simulink library "csc_estimation_lib"  (R2015b)
settings: Solver=ode45  StartTime=0.0  StopTime=10.0  RelTol=1e-3
undefined symbols (not defined in the file): csu_kfo_kalman_filter_output, csu_kfo_kalman_filter_output_lib, est_time_step
libraries: util_info_lib x4, util_common_lib x4, csc_emp_est_mass_props_lib x2, csc_kfl_kalman_filter_lib x2, csc_spc_sensor_processing_lib x2, csu_elk_est_landed_kinematics_lib x2, csu_esf_est_switch_frame_lib x2, util_frame_rotation_lib x2
settings Model: Creator=ianmga  LastModifiedBy=Mark Agbayani
settings DataIOCC: SaveFormat=Array  SignalLoggingSaveFormat=ModelDataLogs
settings OptimizationCC: ExpressionDepthLimit=2147483647
settings DebuggingCC: UnderspecifiedInitializationDetection=Classic  MergeDetectMultiDrivingBlocksExec=none  SolverPrmCheckMsg=warning  FcnCallInpInsideContextMsg=UseLocalSettings  StateNameClashWarn=warning
settings HardwareCC: ProdBitPerPointer=32  ProdLargestAtomicFloat=None  ProdIntDivRoundTo=Undefined  ProdEndianess=Unspecified  ProdWordSize=32  ProdHWDeviceType=32-bit Generic
settings GRTTargetCC: GeneratePreprocessorConditionals=Disable all  CombineOutputUpdateFcns=off  GRTInterface=on
settings ConfigComp: CovModelRefEnable=Off  CovSFcnEnable=off

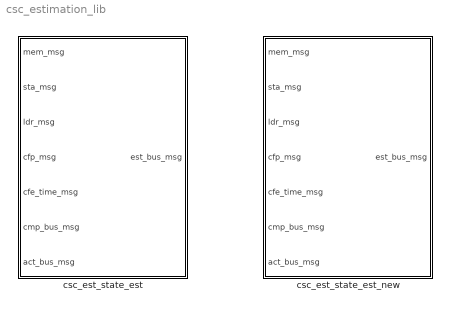
== system csc_estimation_lib ==
  csc_est_state_est : Subsystem  Tag=OFSW; MDL_TICK=CMP_BUS_MSG  TreatAsAtomicUnit=on  SystemSampleTime=est_time_step
  csc_est_state_est_new : Subsystem  Tag=OFSW; MDL_TICK=CMP_BUS_MSG  TreatAsAtomicUnit=on  SystemSampleTime=est_time_step

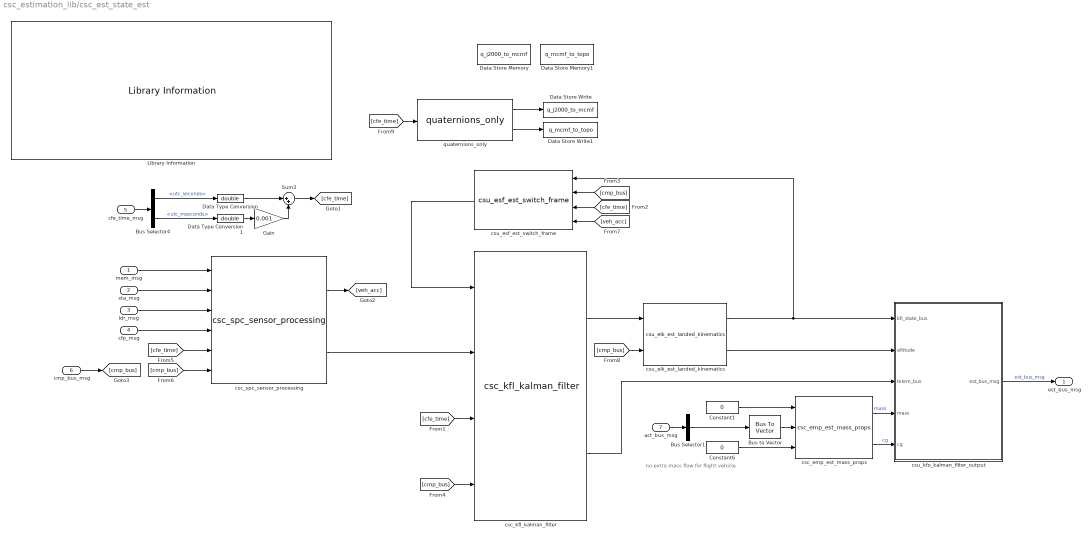
== system csc_estimation_lib/csc_est_state_est ==
  note: no extra mass flow for flight vehicle
  mem_msg : Inport  OutDataTypeStr=Bus: mem_msg
  sta_msg : Inport  Port=2  OutDataTypeStr=Bus: sta_msg
  ldr_msg : Inport  Port=3  OutDataTypeStr=Bus: ldr_msg
  cfp_msg : Inport  Port=4  OutDataTypeStr=Bus: cfp_msg
  cfe_time_msg : Inport  Port=5  OutDataTypeStr=Bus: cfe_time_msg
  cmp_bus_msg : Inport  Port=6  OutDataTypeStr=Bus: cmp_bus_msg
  act_bus_msg : Inport  Port=7  OutDataTypeStr=Bus: act_bus_msg
  Bus Selector1 : BusSelector  OutputSignals=coarse1_time,coarse2_time,coarse3_time,coarse4_time,coarse5_time,coarse6_time,coarse7_time,coarse8_time,coarse9_time,coarse10_time,coarse11_time,coarse12_time,fine1_time,fine2_time,fine3_time,fine4_time,fine5_time,fine6_time,fine7_time,fine8_time,fine9_time,fine10_time,fine11_time,fine12_time,main_thruster_cmd,main_biprop_monoprop  OutputAsBus=on
  Bus Selector4 : BusSelector  OutputSignals=utc_seconds,utc_mseconds
  Bus to Vector : BusToVector
  Constant1 : Constant  Value=0
  Constant6 : Constant  Value=0
  Data Store Memory : DataStoreMemory  DataStoreName=q_j2000_to_mcmf  ReadBeforeWriteMsg=warning  WriteAfterWriteMsg=warning  WriteAfterReadMsg=warning  InitialValue=[0 0 0 1]  OutDataTypeStr=double
  Data Store Memory1 : DataStoreMemory  DataStoreName=q_mcmf_to_topo  ReadBeforeWriteMsg=warning  WriteAfterWriteMsg=warning  WriteAfterReadMsg=warning  InitialValue=[0 0 0 1]  OutDataTypeStr=double
  Data Store Write : DataStoreWrite  DataStoreName=q_j2000_to_mcmf
  Data Store Write1 : DataStoreWrite  DataStoreName=q_mcmf_to_topo
  Data Type Conversion : DataTypeConversion  OutDataTypeStr=double
  Data Type Conversion1 : DataTypeConversion  OutDataTypeStr=double
  Gain : Gain  Gain=0.001
  Library Information : util_info_lib/Library Information  owner='NONE'
  Sum2 : Sum  Inputs=|++
  csc_emp_est_mass_props : csc_emp_est_mass_props_lib/csc_emp_est_mass_props
  csc_kfl_kalman_filter : csc_kfl_kalman_filter_lib/csc_kfl_kalman_filter
  csc_spc_sensor_processing : csc_spc_sensor_processing_lib/csc_spc_sensor_processing
  csu_elk_est_landed_kinematics : csu_elk_est_landed_kinematics_lib/csu_elk_est_landed_kinematics
  csu_esf_est_switch_frame : csu_esf_est_switch_frame_lib/csu_esf_est_switch_frame
  csu_kfo_kalman_filter_output : Subsystem  AncestorBlock=csu_kfo_kalman_filter_output_lib/csu_kfo_kalman_filter_output
  quaternions_only : util_frame_rotation_lib/quaternions_only  SystemSampleTime=-1
  est_bus_msg : Outport  OutDataTypeStr=Bus: est_bus_msg
  wires:
  Bus Selector1/1 -> Bus to Vector/1
  Bus to Vector/1 -> csc_emp_est_mass_props/2
  act_bus_msg/1 -> Bus Selector1/1
  Constant1/1 -> csc_emp_est_mass_props/1
  mem_msg/1 -> csc_spc_sensor_processing/1
  quaternions_only/2 -> Data Store Write1/1
  quaternions_only/1 -> Data Store Write/1
  [cfe_time] -> quaternions_only/1
  csc_spc_sensor_processing/1 -> [veh_acc]
  csc_kfl_kalman_filter/2 -> csu_kfo_kalman_filter_output/3(telem_bus)
  cfe_time_msg/1 -> Bus Selector4/1
  Sum2/1 -> [cfe_time]
  Bus Selector4/2 -> Data Type Conversion1/1  "<utc_mseconds>"
  Bus Selector4/1 -> Data Type Conversion/1  "<utc_seconds>"
  Data Type Conversion/1 -> Sum2/1
  Data Type Conversion1/1 -> Gain/1
  Gain/1 -> Sum2/2
  [veh_acc] -> csu_esf_est_switch_frame/4
  csu_elk_est_landed_kinematics/2 -> csu_kfo_kalman_filter_output/2(altitude)
  [cmp_bus] -> csu_elk_est_landed_kinematics/2
  csu_elk_est_landed_kinematics/1 -> csu_kfo_kalman_filter_output/1(kfl_state_bus), csu_esf_est_switch_frame/1
  csc_kfl_kalman_filter/1 -> csu_elk_est_landed_kinematics/1
  csc_spc_sensor_processing/2 -> csc_kfl_kalman_filter/2
  [cmp_bus] -> csc_spc_sensor_processing/6
  [cfe_time] -> csc_spc_sensor_processing/5
  ldr_msg/1 -> csc_spc_sensor_processing/3
  sta_msg/1 -> csc_spc_sensor_processing/2
  [cmp_bus] -> csc_kfl_kalman_filter/4
  [cfe_time] -> csc_kfl_kalman_filter/3
  [cmp_bus] -> csu_esf_est_switch_frame/2
  [cfe_time] -> csu_esf_est_switch_frame/3
  cmp_bus_msg/1 -> [cmp_bus]
  csu_esf_est_switch_frame/1 -> csc_kfl_kalman_filter/1
  csu_kfo_kalman_filter_output/1(est_bus_msg) -> est_bus_msg/1  "est_bus_msg"
  cfp_msg/1 -> csc_spc_sensor_processing/4
  Constant6/1 -> csc_emp_est_mass_props/3
  csc_emp_est_mass_props/2 -> csu_kfo_kalman_filter_output/5(cg)  "cg"
  csc_emp_est_mass_props/1 -> csu_kfo_kalman_filter_output/4(mass)  "mass"

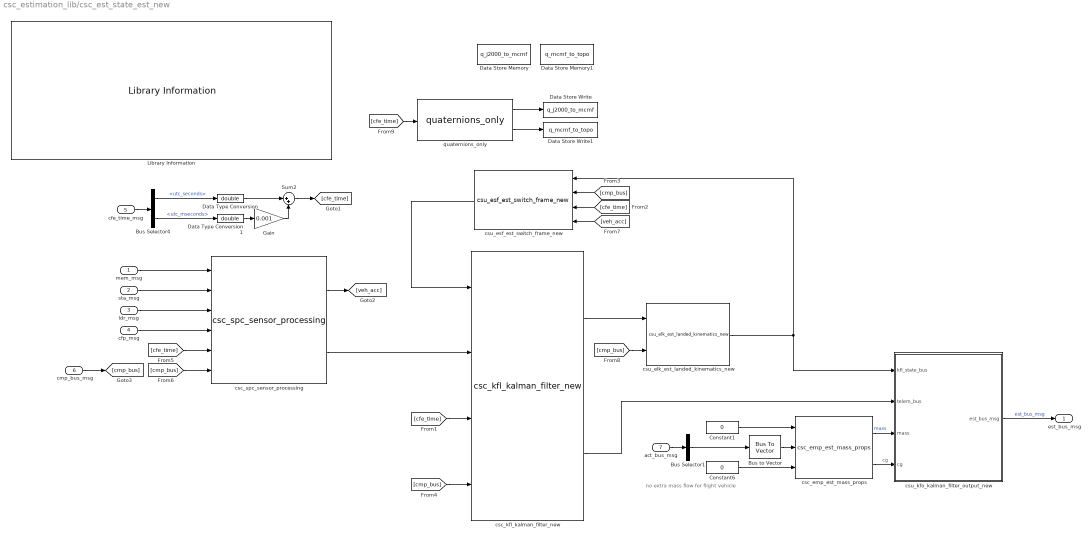
== system csc_estimation_lib/csc_est_state_est_new ==
  note: no extra mass flow for flight vehicle
  mem_msg : Inport  OutDataTypeStr=Bus: mem_msg
  sta_msg : Inport  Port=2  OutDataTypeStr=Bus: sta_msg
  ldr_msg : Inport  Port=3  OutDataTypeStr=Bus: ldr_msg
  cfp_msg : Inport  Port=4  OutDataTypeStr=Bus: cfp_msg
  cfe_time_msg : Inport  Port=5  OutDataTypeStr=Bus: cfe_time_msg
  cmp_bus_msg : Inport  Port=6  OutDataTypeStr=Bus: cmp_bus_msg
  act_bus_msg : Inport  Port=7  OutDataTypeStr=Bus: act_bus_msg
  Bus Selector1 : BusSelector  OutputSignals=coarse1_time,coarse2_time,coarse3_time,coarse4_time,coarse5_time,coarse6_time,coarse7_time,coarse8_time,coarse9_time,coarse10_time,coarse11_time,coarse12_time,fine1_time,fine2_time,fine3_time,fine4_time,fine5_time,fine6_time,fine7_time,fine8_time,fine9_time,fine10_time,fine11_time,fine12_time,main_thruster_cmd,main_biprop_monoprop  OutputAsBus=on
  Bus Selector4 : BusSelector  OutputSignals=utc_seconds,utc_mseconds
  Bus to Vector : BusToVector
  Constant1 : Constant  Value=0
  Constant6 : Constant  Value=0
  Data Store Memory : DataStoreMemory  DataStoreName=q_j2000_to_mcmf  ReadBeforeWriteMsg=warning  WriteAfterWriteMsg=warning  WriteAfterReadMsg=warning  InitialValue=[0 0 0 1]  OutDataTypeStr=double
  Data Store Memory1 : DataStoreMemory  DataStoreName=q_mcmf_to_topo  ReadBeforeWriteMsg=warning  WriteAfterWriteMsg=warning  WriteAfterReadMsg=warning  InitialValue=[0 0 0 1]  OutDataTypeStr=double
  Data Store Write : DataStoreWrite  DataStoreName=q_j2000_to_mcmf
  Data Store Write1 : DataStoreWrite  DataStoreName=q_mcmf_to_topo
  Data Type Conversion : DataTypeConversion  OutDataTypeStr=double
  Data Type Conversion1 : DataTypeConversion  OutDataTypeStr=double
  Gain : Gain  Gain=0.001
  Library Information : util_info_lib/Library Information  owner='NONE'
  Sum2 : Sum  Inputs=|++
  csc_emp_est_mass_props : csc_emp_est_mass_props_lib/csc_emp_est_mass_props
  csc_kfl_kalman_filter_new : csc_kfl_kalman_filter_lib/csc_kfl_kalman_filter_new
  csc_spc_sensor_processing : csc_spc_sensor_processing_lib/csc_spc_sensor_processing
  csu_elk_est_landed_kinematics_new : csu_elk_est_landed_kinematics_lib/csu_elk_est_landed_kinematics_new
  csu_esf_est_switch_frame_new : csu_esf_est_switch_frame_lib/csu_esf_est_switch_frame_new
  csu_kfo_kalman_filter_output_new : Subsystem
  quaternions_only : util_frame_rotation_lib/quaternions_only  SystemSampleTime=-1
  est_bus_msg : Outport  OutDataTypeStr=Bus: est_bus_msg
  wires:
  Bus Selector1/1 -> Bus to Vector/1
  Bus to Vector/1 -> csc_emp_est_mass_props/2
  act_bus_msg/1 -> Bus Selector1/1
  Constant1/1 -> csc_emp_est_mass_props/1
  mem_msg/1 -> csc_spc_sensor_processing/1
  quaternions_only/2 -> Data Store Write1/1
  quaternions_only/1 -> Data Store Write/1
  [cfe_time] -> quaternions_only/1
  csc_spc_sensor_processing/1 -> [veh_acc]
  csc_kfl_kalman_filter_new/2 -> csu_kfo_kalman_filter_output_new/2(telem_bus)
  cfe_time_msg/1 -> Bus Selector4/1
  Sum2/1 -> [cfe_time]
  Bus Selector4/2 -> Data Type Conversion1/1  "<utc_mseconds>"
  Bus Selector4/1 -> Data Type Conversion/1  "<utc_seconds>"
  Data Type Conversion/1 -> Sum2/1
  Data Type Conversion1/1 -> Gain/1
  Gain/1 -> Sum2/2
  [veh_acc] -> csu_esf_est_switch_frame_new/4
  [cmp_bus] -> csu_elk_est_landed_kinematics_new/2
  csu_elk_est_landed_kinematics_new/1 -> csu_kfo_kalman_filter_output_new/1(kfl_state_bus), csu_esf_est_switch_frame_new/1
  csc_kfl_kalman_filter_new/1 -> csu_elk_est_landed_kinematics_new/1
  csc_spc_sensor_processing/2 -> csc_kfl_kalman_filter_new/2
  [cmp_bus] -> csc_spc_sensor_processing/6
  [cfe_time] -> csc_spc_sensor_processing/5
  ldr_msg/1 -> csc_spc_sensor_processing/3
  sta_msg/1 -> csc_spc_sensor_processing/2
  [cmp_bus] -> csc_kfl_kalman_filter_new/4
  [cfe_time] -> csc_kfl_kalman_filter_new/3
  [cmp_bus] -> csu_esf_est_switch_frame_new/2
  [cfe_time] -> csu_esf_est_switch_frame_new/3
  cmp_bus_msg/1 -> [cmp_bus]
  csu_esf_est_switch_frame_new/1 -> csc_kfl_kalman_filter_new/1
  csu_kfo_kalman_filter_output_new/1(est_bus_msg) -> est_bus_msg/1  "est_bus_msg"
  cfp_msg/1 -> csc_spc_sensor_processing/4
  Constant6/1 -> csc_emp_est_mass_props/3
  csc_emp_est_mass_props/2 -> csu_kfo_kalman_filter_output_new/4(cg)  "cg"
  csc_emp_est_mass_props/1 -> csu_kfo_kalman_filter_output_new/3(mass)  "mass"

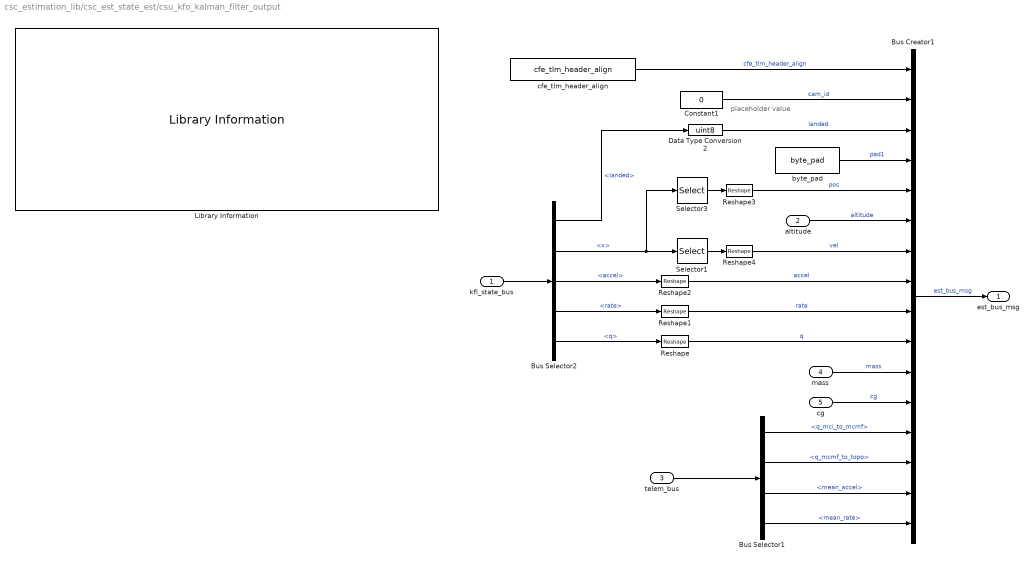
== system csc_estimation_lib/csc_est_state_est/csu_kfo_kalman_filter_output ==
  note: placeholder value
  kfl_state_bus : Inport
  altitude : Inport  Port=2
  telem_bus : Inport  Port=3
  mass : Inport  Port=4
  cg : Inport  Port=5
  Bus Creator1 : BusCreator  Inputs=16  OutDataTypeStr=Bus: est_bus_msg  NonVirtualBus=on
  Bus Selector1 : BusSelector  OutputSignals=q_mci_to_mcmf,q_mcmf_to_topo,mean_accel,mean_rate
  Bus Selector2 : BusSelector  OutputSignals=landed,x,accel,rate,q
  Constant1 : Constant  Value=0  OutDataTypeStr=uint8
  Data Type Conversion2 : DataTypeConversion  OutDataTypeStr=uint8
  Library Information : util_info_lib/Library Information  owner='escrane'
  Reshape{,1..4} (5 alike) : Reshape
  Selector1 : Selector  InputPortWidth=kfl_n_state  IndexOptions=Index vector (dialog)  Indices=kfl_vel_index  OutputSizes=1
  Selector3 : Selector  InputPortWidth=kfl_n_state  IndexOptions=Index vector (dialog)  Indices=kfl_pos_index  OutputSizes=1
  byte_pad : util_common_lib/byte_pad  n_bytes=2
  cfe_tlm_header_align : util_common_lib/cfe_tlm_header_align
  est_bus_msg : Outport
  wires:
  altitude/1 -> Bus Creator1/6  "altitude"
  Data Type Conversion2/1 -> Bus Creator1/3  "landed"
  Selector3/1 -> Reshape3/1
  Reshape3/1 -> Bus Creator1/5  "pos"
  Reshape4/1 -> Bus Creator1/7  "vel"
  Reshape1/1 -> Bus Creator1/9  "rate"
  Reshape/1 -> Bus Creator1/10  "q"
  Bus Selector2/2 -> Selector3/1, Selector1/1  "<x>"
  Selector1/1 -> Reshape4/1
  Bus Selector2/3 -> Reshape2/1  "<accel>"
  Bus Selector2/4 -> Reshape1/1  "<rate>"
  Bus Selector2/5 -> Reshape/1  "<q>"
  Bus Creator1/1 -> est_bus_msg/1  "est_bus_msg"
  Reshape2/1 -> Bus Creator1/8  "accel"
  Constant1/1 -> Bus Creator1/2  "cam_id"
  byte_pad/1 -> Bus Creator1/4  "pad1"
  Bus Selector2/1 -> Data Type Conversion2/1  "<landed>"
  cfe_tlm_header_align/1 -> Bus Creator1/1  "cfe_tlm_header_align"
  kfl_state_bus/1 -> Bus Selector2/1
  mass/1 -> Bus Creator1/11  "mass"
  cg/1 -> Bus Creator1/12  "cg"
  telem_bus/1 -> Bus Selector1/1
  Bus Selector1/2 -> Bus Creator1/14  "<q_mcmf_to_topo>"
  Bus Selector1/1 -> Bus Creator1/13  "<q_mci_to_mcmf>"
  Bus Selector1/3 -> Bus Creator1/15  "<mean_accel>"
  Bus Selector1/4 -> Bus Creator1/16  "<mean_rate>"

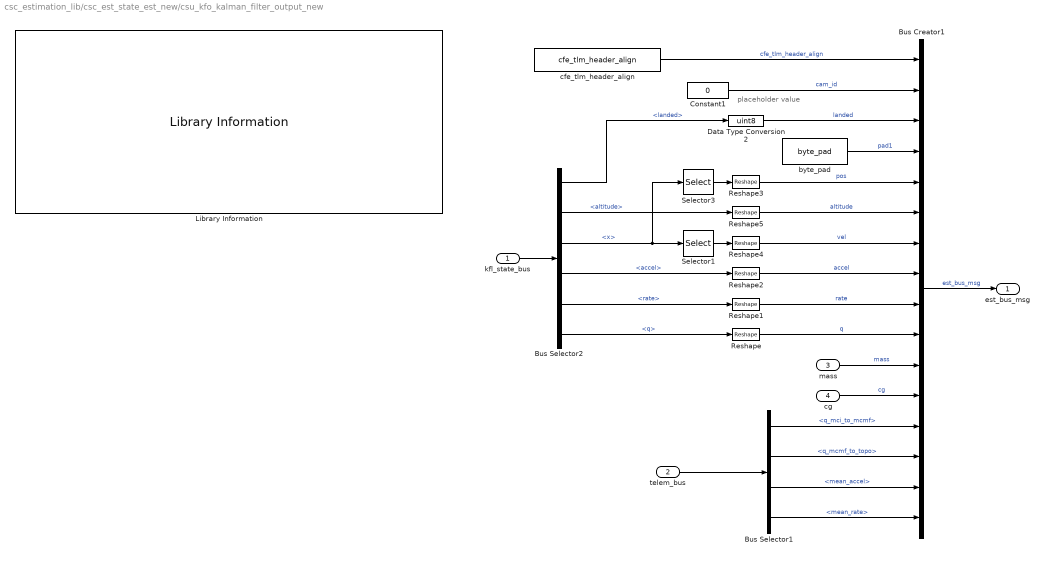
== system csc_estimation_lib/csc_est_state_est_new/csu_kfo_kalman_filter_output_new ==
  note: placeholder value
  kfl_state_bus : Inport
  telem_bus : Inport  Port=2
  mass : Inport  Port=3
  cg : Inport  Port=4
  Bus Creator1 : BusCreator  Inputs=16  OutDataTypeStr=Bus: est_bus_msg  NonVirtualBus=on
  Bus Selector1 : BusSelector  OutputSignals=q_mci_to_mcmf,q_mcmf_to_topo,mean_accel,mean_rate
  Bus Selector2 : BusSelector  OutputSignals=landed,altitude,x,accel,rate,q
  Constant1 : Constant  Value=0  OutDataTypeStr=uint8
  Data Type Conversion2 : DataTypeConversion  OutDataTypeStr=uint8
  Library Information : util_info_lib/Library Information  owner='escrane'
  Reshape{,1..5} (6 alike) : Reshape
  Selector1 : Selector  InputPortWidth=kfl_n_state  IndexOptions=Index vector (dialog)  Indices=kfl_vel_index  OutputSizes=1
  Selector3 : Selector  InputPortWidth=kfl_n_state  IndexOptions=Index vector (dialog)  Indices=kfl_pos_index  OutputSizes=1
  byte_pad : util_common_lib/byte_pad  n_bytes=2
  cfe_tlm_header_align : util_common_lib/cfe_tlm_header_align
  est_bus_msg : Outport
  wires:
  Reshape5/1 -> Bus Creator1/6  "altitude"
  Bus Selector1/4 -> Bus Creator1/16  "<mean_rate>"
  Bus Selector1/3 -> Bus Creator1/15  "<mean_accel>"
  Bus Selector1/1 -> Bus Creator1/13  "<q_mci_to_mcmf>"
  Bus Selector1/2 -> Bus Creator1/14  "<q_mcmf_to_topo>"
  telem_bus/1 -> Bus Selector1/1
  cg/1 -> Bus Creator1/12  "cg"
  mass/1 -> Bus Creator1/11  "mass"
  kfl_state_bus/1 -> Bus Selector2/1
  cfe_tlm_header_align/1 -> Bus Creator1/1  "cfe_tlm_header_align"
  Bus Selector2/1 -> Data Type Conversion2/1  "<landed>"
  byte_pad/1 -> Bus Creator1/4  "pad1"
  Constant1/1 -> Bus Creator1/2  "cam_id"
  Reshape2/1 -> Bus Creator1/8  "accel"
  Bus Creator1/1 -> est_bus_msg/1  "est_bus_msg"
  Bus Selector2/6 -> Reshape/1  "<q>"
  Bus Selector2/5 -> Reshape1/1  "<rate>"
  Bus Selector2/4 -> Reshape2/1  "<accel>"
  Selector1/1 -> Reshape4/1
  Bus Selector2/3 -> Selector1/1, Selector3/1  "<x>"
  Reshape/1 -> Bus Creator1/10  "q"
  Reshape1/1 -> Bus Creator1/9  "rate"
  Reshape4/1 -> Bus Creator1/7  "vel"
  Reshape3/1 -> Bus Creator1/5  "pos"
  Selector3/1 -> Reshape3/1
  Data Type Conversion2/1 -> Bus Creator1/3  "landed"
  Bus Selector2/2 -> Reshape5/1  "<altitude>"
